simulink model "SystemModel"  (R2017a)
settings: Solver=ode45  StartTime=0.0  StopTime=10.0  RelTol=1e-3
model workspace: external: MATLAB File C:\Users\Josh\jmccread@umich.edu\UMD\ECE560\Term Project\ECE560\CompensatorDesignTool.m (data not in the file)
values from neighbouring files (symbols this model uses):
  g = 9.8    [CartPole.m]    (also in CompensatorDesignTool.m; DisturbanceRejectionDesignTool.m; LQRDesignTool.m; LinearizationWork.m)
  l = 0.5    [CartPole.m]    (also in CompensatorDesignTool.m; DisturbanceRejectionDesignTool.m; LQRDesignTool.m; LinearizationWork.m)
  L = (I + m*l^2)/(m*l)    (= 1)    [CartPole.m]    (also in CartPoleLinearSystem.m = (I + m*l^2)/(m*l); CartPoleSystem.m = (I + m*l^2)/(m*l); CartPoleSystemObs.m = (I + m*l^2)/(m*l); CompensatorDesignTool.m)
  m = 0.1    [CartPole.m]    (also in CompensatorDesignTool.m; DisturbanceRejectionDesignTool.m; LQRDesignTool.m; LinearizationWork.m)
  Mt = M + m    (= 2.1)    [CartPole.m]    (also in CartPoleLinearSystem.m = M + m; CartPoleSystem.m = M + m; CartPoleSystemObs.m = M + m; CompensatorDesignTool.m)
undefined symbols (not defined in the file or in its folder): K2, K3, K4, x_0_1, x_0_2, x_0_3, x_0_4, x_d_1, x_d_2, x_d_3, x_d_4
settings Model: Creator=Josh  LastModifiedBy=Josh

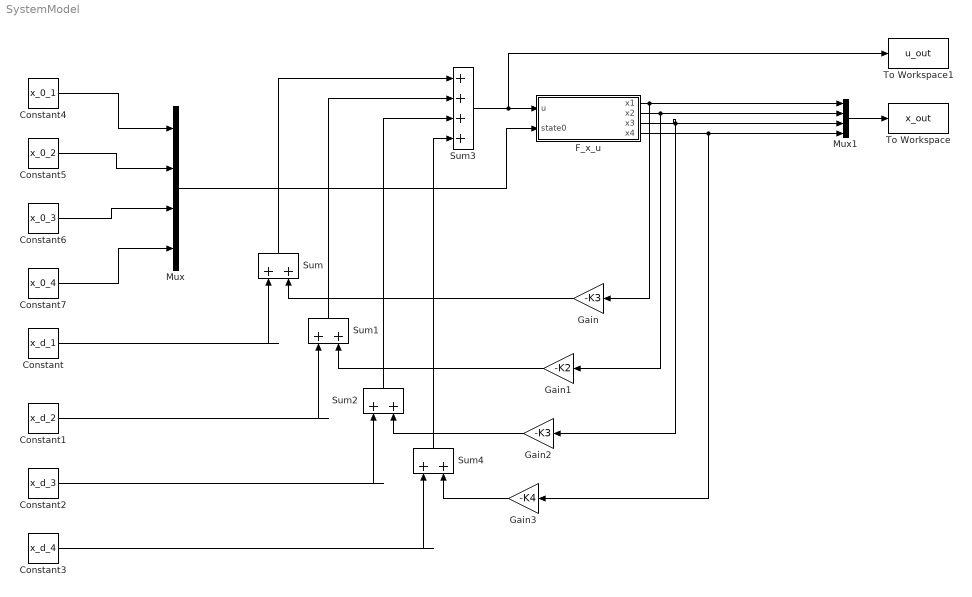
== system SystemModel ==
  Constant : Constant  Value=x_d_1
  Constant1 : Constant  Value=x_d_2
  Constant2 : Constant  Value=x_d_3
  Constant3 : Constant  Value=x_d_4
  Constant4 : Constant  Value=x_0_1
  Constant5 : Constant  Value=x_0_2
  Constant6 : Constant  Value=x_0_3
  Constant7 : Constant  Value=x_0_4
  F_x_u : Subsystem
  Gain : Gain  Gain=-K3
  Gain1 : Gain  Gain=-K2
  Gain2 : Gain  Gain=-K3
  Gain3 : Gain  Gain=-K4
  Mux : Mux
  Mux1 : Mux
  Sum{,1..2,4} (4 alike) : Sum  Inputs=|++
  Sum3 : Sum  Inputs=4
  To Workspace : ToWorkspace  VariableName=x_out  SaveFormat=Timeseries  SampleTime=-1
  To Workspace1 : ToWorkspace  VariableName=u_out  SaveFormat=Timeseries  SampleTime=-1
  wires:
  Mux/1 -> F_x_u/2(state0)
  F_x_u/1(x1) -> Mux1/1, Gain/1
  F_x_u/2(x2) -> Mux1/2, Gain1/1
  F_x_u/3(x3) -> Mux1/3, Gain2/1
  F_x_u/4(x4) -> Mux1/4, Gain3/1
  Gain/1 -> Sum/2
  Sum/1 -> Sum3/1
  Gain1/1 -> Sum1/2
  Constant1/1 -> Sum1/1
  Sum1/1 -> Sum3/2
  Gain2/1 -> Sum2/2
  Constant2/1 -> Sum2/1
  Sum2/1 -> Sum3/3
  Gain3/1 -> Sum4/2
  Constant3/1 -> Sum4/1
  Sum4/1 -> Sum3/4
  Sum3/1 -> To Workspace1/1, F_x_u/1("u ")
  Constant/1 -> Sum/1
  Constant4/1 -> Mux/1
  Constant5/1 -> Mux/2
  Constant6/1 -> Mux/3
  Constant7/1 -> Mux/4
  Mux1/1 -> To Workspace/1

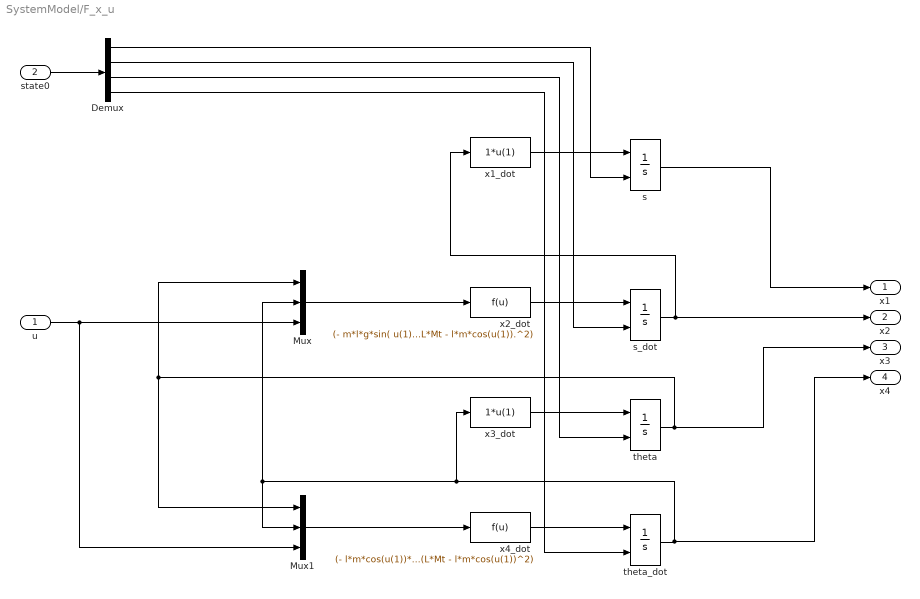
== system SystemModel/F_x_u ==
  "u " : Inport
  state0 : Inport  Port=2
  Demux : Demux
  Mux : Mux  Inputs=3
  Mux1 : Mux  Inputs=3
  s : Integrator  InitialConditionSource=external  ContinuousStateAttributes='pos_dot'
  s_dot : Integrator  InitialConditionSource=external  ContinuousStateAttributes='pos_dot'
  theta : Integrator  InitialConditionSource=external  ContinuousStateAttributes='theta'
  theta_dot : Integrator  InitialConditionSource=external  ContinuousStateAttributes='theta'
  x1_dot : Fcn  Expr=1*u(1)
  x2_dot : Fcn  Expr=(- m*l*g*sin( u(1)).*cos(u(1)) + m*l*L*sin(u(1)).*u(2).^2)/(Mt*L - m*l*(cos(u(1)).^2)) +(L*u(3))/(L*Mt - l*m*cos(u(1)).^2)
  x3_dot : Fcn  Expr=1*u(1)
  x4_dot : Fcn  Expr=(- l*m*cos(u(1))*sin(u(3))*u(2)^2 + Mt*g*sin(u(1)))/(L*Mt - l*m*cos(u(1))^2) - (u(3)*cos(u(1)))/(L*Mt - l*m*cos(u(1))^2)
  x1 : Outport
  x2 : Outport  Port=2
  x3 : Outport  Port=3
  x4 : Outport  Port=4
  wires:
  Mux1/1 -> x4_dot/1
  x1_dot/1 -> s/1
  theta_dot/1 -> x4/1, Mux/2, Mux1/2, x3_dot/1
  theta/1 -> x3/1, Mux1/1, Mux/1
  "u "/1 -> Mux1/3, Mux/3
  Mux/1 -> x2_dot/1
  x4_dot/1 -> theta_dot/1
  Demux/4 -> theta_dot/2
  s_dot/1 -> x2/1, x1_dot/1
  Demux/2 -> s_dot/2
  x3_dot/1 -> theta/1
  x2_dot/1 -> s_dot/1
  Demux/1 -> s/2
  Demux/3 -> theta/2
  s/1 -> x1/1
  state0/1 -> Demux/1
